simulink model "unitdelay_test"  (Simulink 9.0)
settings: Solver=FixedStepAuto  StartTime=0.0  StopTime=10.0  FixedStep=1.000000  RelTol=1e-3  EnableMultiTasking=on
settings Model: SuppressorTable=22 serialization::archive 11 0 6 0 0 0 0 0  Creator=arnaud  LastModifiedBy=hbourbou
settings DataIOCC: LimitDataPoints=on  SaveFormat=Structure  SignalLoggingSaveFormat=ModelDataLogs
settings OptimizationCC: ExpressionDepthLimit=2147483647
settings DebuggingCC: SolverPrmCheckMsg=warning  FcnCallInpInsideContextMsg=warning  StateNameClashWarn=warning  StrictBusMsg=Warning
settings GRTTargetCC: CombineOutputUpdateFcns=off  GRTInterface=on

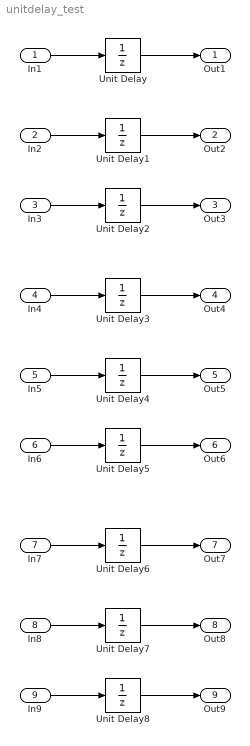
== system unitdelay_test ==
  In1 : Inport  OutDataTypeStr=double  PortDimensions=1
  In2 : Inport  Port=2  OutDataTypeStr=double  PortDimensions=1
  In3 : Inport  Port=3  PortDimensions=1
  In4 : Inport  Port=4  OutDataTypeStr=int8  PortDimensions=1
  In5 : Inport  Port=5  OutDataTypeStr=int8  PortDimensions=1
  In6 : Inport  Port=6  OutDataTypeStr=int8  PortDimensions=1
  In7 : Inport  Port=7  OutDataTypeStr=boolean  PortDimensions=1
  In8 : Inport  Port=8  OutDataTypeStr=boolean  PortDimensions=1
  In9 : Inport  Port=9  OutDataTypeStr=boolean  PortDimensions=1
  Unit Delay : UnitDelay
  Unit Delay1 : UnitDelay  InitialCondition=0.0
  Unit Delay2 : UnitDelay  InitialCondition=true
  Unit Delay3 : UnitDelay
  Unit Delay4 : UnitDelay  InitialCondition=0.0
  Unit Delay5 : UnitDelay  InitialCondition=true
  Unit Delay6 : UnitDelay
  Unit Delay7 : UnitDelay  InitialCondition=0.0
  Unit Delay8 : UnitDelay  InitialCondition=true
  Out1 : Outport
  Out2 : Outport  Port=2
  Out3 : Outport  Port=3
  Out4 : Outport  Port=4
  Out5 : Outport  Port=5
  Out6 : Outport  Port=6
  Out7 : Outport  Port=7
  Out8 : Outport  Port=8
  Out9 : Outport  Port=9
  wires:
  In1/1 -> Unit Delay/1
  Unit Delay/1 -> Out1/1
  In2/1 -> Unit Delay1/1
  Unit Delay1/1 -> Out2/1
  In3/1 -> Unit Delay2/1
  Unit Delay2/1 -> Out3/1
  In4/1 -> Unit Delay3/1
  Unit Delay3/1 -> Out4/1
  In5/1 -> Unit Delay4/1
  Unit Delay4/1 -> Out5/1
  In6/1 -> Unit Delay5/1
  Unit Delay5/1 -> Out6/1
  In7/1 -> Unit Delay6/1
  Unit Delay6/1 -> Out7/1
  In8/1 -> Unit Delay7/1
  Unit Delay7/1 -> Out8/1
  In9/1 -> Unit Delay8/1
  Unit Delay8/1 -> Out9/1
